simulink model "ch7_2nd_eye_OL"  (R2017a)
settings: Solver=ode3  StartTime=0.0  StopTime=0.2  FixedStep=.001  MaxStep=.002  RelTol=1e-3  EnableMultiTasking=on
settings Model: Creator=wintersj  LastModifiedBy=wintersj
settings DataIOCC: LimitDataPoints=on  SaveFormat=Array  SignalLoggingSaveFormat=ModelDataLogs
settings OptimizationCC: ExpressionDepthLimit=2147483647  LifeSpan=inf
settings DebuggingCC: UnderspecifiedInitializationDetection=Classic  MergeDetectMultiDrivingBlocksExec=none  MaxConsecutiveZCsMsg=none  SolverPrmCheckMsg=warning  FcnCallInpInsideContextMsg=warning  StateNameClashWarn=warning  SFUnexpectedBacktrackingDiag=warning  SFNoUnconditionalDefaultTransitionDiag=warning  SFExecutionAtInitializationDiag=none
settings HardwareCC: ProdBitPerPointer=32  ProdBitPerSizeT=32  ProdBitPerPtrDiffT=32  ProdLargestAtomicFloat=None  ProdIntDivRoundTo=Undefined  ProdEndianess=Unspecified  ProdWordSize=32  ProdHWDeviceType=32-bit Generic
settings ModelReferenceCC: PropagateSignalLabelsOutOfModel=off
settings GRTTargetCC: TargetLangStandard=C89/C90 (ANSI)  GeneratePreprocessorConditionals=Disable all  CombineOutputUpdateFcns=off  GRTInterface=on
settings ConfigComp: CovMetricSettings=dw  CovHtmlReporting=on  CovSaveCumulativeToWorkspaceVar=on  CovSaveSingleToWorkspaceVar=on  CovExternalEMLEnable=off

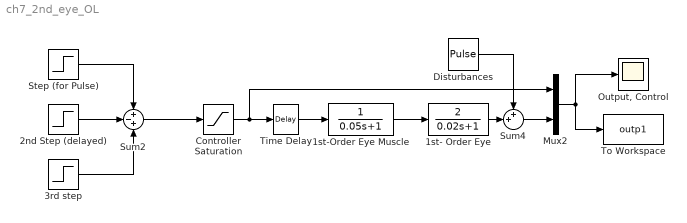
== system ch7_2nd_eye_OL ==
  "1st- Order Eye " : TransferFcn  Numerator=[2]  Denominator=[0.02 1]
  1st-Order Eye Muscle : TransferFcn  Denominator=[0.05 1]
  2nd Step (delayed) : Step  Time=.03  Before=0.01  After=0.8  SampleTime=0
  "3rd step " : Step  Time=0.1  After=0  SampleTime=0
  Controller Saturation : Saturate  UpperLimit=1  LowerLimit=-1
  Disturbances : DiscretePulseGenerator  PulseType=Time based  Amplitude=0  Period=0.3  PulseWidth=50  PhaseDelay=0.1
  Mux2 : Mux  Inputs=2
  "Output, Control" : Scope
  Step (for Pulse) : Step  Time=0.01  Before=0.01  SampleTime=0
  Sum2 : Sum  Inputs=+-+
  Sum4 : Sum  Inputs=++|
  Time Delay : TransportDelay  DelayTime=0.01
  To Workspace : ToWorkspace  VariableName=outp1  SampleTime=-1
  wires:
  Controller Saturation/1 -> Time Delay/1, Mux2/1
  "1st- Order Eye "/1 -> Sum4/2
  Sum4/1 -> Mux2/2
  Mux2/1 -> To Workspace/1, "Output, Control"/1
  Disturbances/1 -> Sum4/1
  Time Delay/1 -> 1st-Order Eye Muscle/1
  1st-Order Eye Muscle/1 -> "1st- Order Eye "/1
  Step (for Pulse)/1 -> Sum2/1
  2nd Step (delayed)/1 -> Sum2/2
  Sum2/1 -> Controller Saturation/1
  "3rd step "/1 -> Sum2/3
